simulink model "Prac04_1_g"  (R2015a)
settings: Solver=ode45  StartTime=0.0  StopTime=8  RelTol=1e-3
libraries: dspsrcs4 x4, dsparch4 x2, dspsigops x2
settings Model: Creator=Josemi  LastModifiedBy=Josemi

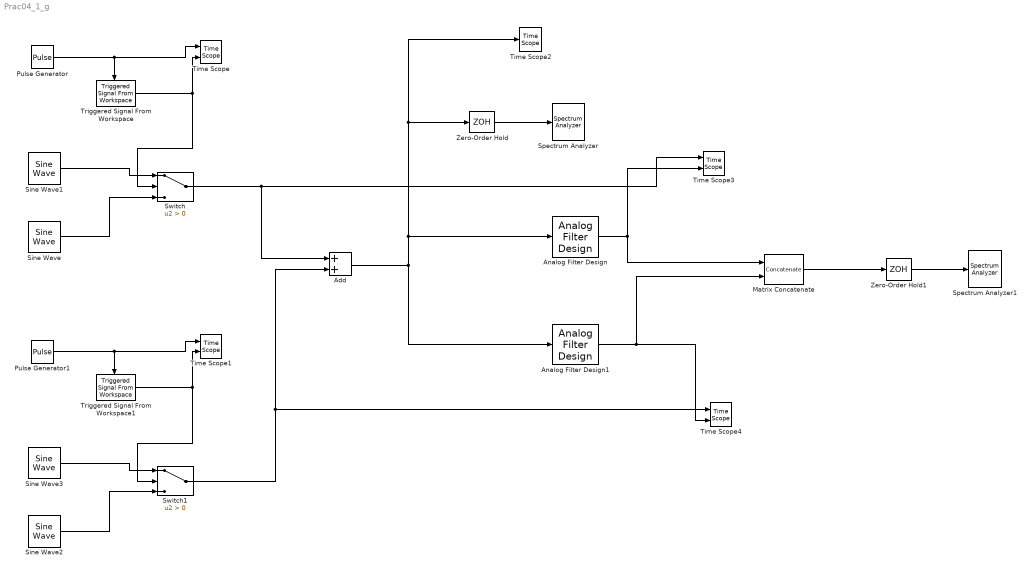
== system Prac04_1_g ==
  Add : Sum
  Analog Filter Design : dsparch4/Analog Filter Design  method=Butterworth  filttype=Bandpass  N=8  Wlo=2*pi*18  Whi=2*pi*22  Rp=2  Rs=40
  Analog Filter Design1 : dsparch4/Analog Filter Design  method=Butterworth  filttype=Bandpass  N=8  Wlo=2*pi*48  Whi=2*pi*52  Rp=2  Rs=40
  Matrix Concatenate : Concatenate  Mode=Multidimensional array  ConcatenateDimension=2
  Pulse Generator : DiscretePulseGenerator  PulseType=Time based  Amplitude=0.5  Period=0.5  PulseWidth=50
  Pulse Generator1 : DiscretePulseGenerator  PulseType=Time based  Amplitude=0.5  Period=0.5  PulseWidth=50
  Sine Wave : dspsrcs4/Sine Wave  Amplitude=0  Frequency=20  Phase=0  SampleMode=Discrete  OutComplex=Real  CompMethod=Trigonometric fcn  TableSize=Speed  SampleTime=0.0025  SamplesPerFrame=1  ResetState=Restart at time zero  dataType=double  wordLen=16  udDataType=sfix(16)  fracBitsMode=Best precision  numFracBits=15  OutDataTypeStr=double  LastOutDataTypeStr=double
  Sine Wave1 : dspsrcs4/Sine Wave  Amplitude=2  Frequency=20  Phase=0  SampleMode=Discrete  OutComplex=Real  CompMethod=Trigonometric fcn  TableSize=Speed  SampleTime=0.0025  SamplesPerFrame=1  ResetState=Restart at time zero  dataType=double  wordLen=16  udDataType=sfix(16)  fracBitsMode=Best precision  numFracBits=15  OutDataTypeStr=double  LastOutDataTypeStr=double
  Sine Wave2 : dspsrcs4/Sine Wave  Amplitude=0  Frequency=50  Phase=0  SampleMode=Discrete  OutComplex=Real  CompMethod=Trigonometric fcn  TableSize=Speed  SampleTime=0.0025  SamplesPerFrame=1  ResetState=Restart at time zero  dataType=double  wordLen=16  udDataType=sfix(16)  fracBitsMode=Best precision  numFracBits=15  OutDataTypeStr=double  LastOutDataTypeStr=double
  Sine Wave3 : dspsrcs4/Sine Wave  Amplitude=2  Frequency=50  Phase=0  SampleMode=Discrete  OutComplex=Real  CompMethod=Trigonometric fcn  TableSize=Speed  SampleTime=0.0025  SamplesPerFrame=1  ResetState=Restart at time zero  dataType=double  wordLen=16  udDataType=sfix(16)  fracBitsMode=Best precision  numFracBits=15  OutDataTypeStr=double  LastOutDataTypeStr=double
  Spectrum Analyzer : SpectrumAnalyzer
  Spectrum Analyzer1 : SpectrumAnalyzer
  Switch : Switch  Criteria=u2 > Threshold
  Switch1 : Switch  Criteria=u2 > Threshold
  Time Scope{,1,3..4} (4 alike) : TimeScope  DefaultConfigurationName=spbscopes.TimeScopeBlockCfg  NumInputPorts=2
  Time Scope2 : TimeScope  DefaultConfigurationName=spbscopes.TimeScopeBlockCfg
  Triggered Signal From Workspace : dspsigops/Triggered Signal From Workspace  Signal=[0 1 0 1 0 0 0 1 1 1 0 1 0 0 0 0]  TriggerType=Rising edge  ic=0  SamplesPerFrame=1  OutputAfterFinalValue=Setting to zero
  Triggered Signal From Workspace1 : dspsigops/Triggered Signal From Workspace  Signal=[0 1 0 1 0 0 1 1 0 1 1 1 0 1 0 1]  TriggerType=Rising edge  ic=0  SamplesPerFrame=1  OutputAfterFinalValue=Setting to zero
  Zero-Order Hold : ZeroOrderHold  SampleTime=0.0025
  Zero-Order Hold1 : ZeroOrderHold  SampleTime=0.0025
  wires:
  Pulse Generator/1 -> Time Scope/1, Triggered Signal From Workspace/Trigger
  Sine Wave1/1 -> Switch/1
  Sine Wave/1 -> Switch/3
  Triggered Signal From Workspace/1 -> Switch/2, Time Scope/2
  Pulse Generator1/1 -> Time Scope1/1, Triggered Signal From Workspace1/Trigger
  Sine Wave3/1 -> Switch1/1
  Sine Wave2/1 -> Switch1/3
  Triggered Signal From Workspace1/1 -> Switch1/2, Time Scope1/2
  Switch/1 -> Time Scope3/1, Add/1
  Switch1/1 -> Time Scope4/1, Add/2
  Zero-Order Hold/1 -> Spectrum Analyzer/1
  Add/1 -> Analog Filter Design1/1, Analog Filter Design/1, Time Scope2/1, Zero-Order Hold/1
  Analog Filter Design/1 -> Matrix Concatenate/1, Time Scope3/2
  Analog Filter Design1/1 -> Matrix Concatenate/2, Time Scope4/2
  Zero-Order Hold1/1 -> Spectrum Analyzer1/1
  Matrix Concatenate/1 -> Zero-Order Hold1/1
